simulink model "inertia_sensor"  (R2024b)
settings: Solver=VariableStepAuto  StartTime=0.0  StopTime=10.0  RelTol=1e-3
libraries: nesl_utility x7, sm_lib x6
settings Model: Creator=tarak  LastModifiedBy=tarak

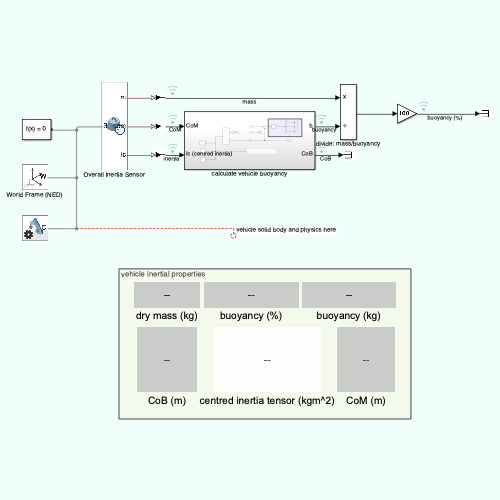
[thumbnail: Simulink's stored preview of the top-level diagram]
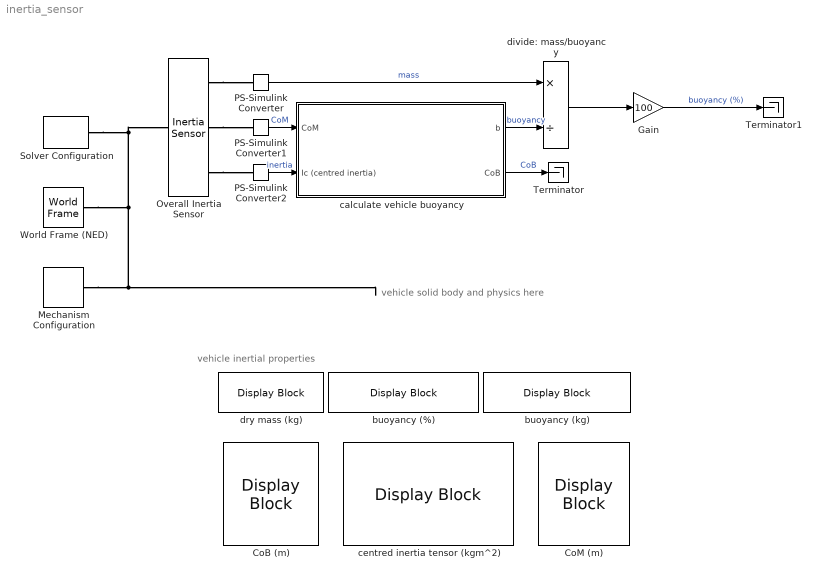
== system inertia_sensor ==
  note: vehicle inertial properties
  note: vehicle solid body and physics here
  CoB (m) : DisplayBlock  LabelPosition=Hide  Transparency=1
  CoM (m) : DisplayBlock  LabelPosition=Hide  Transparency=1
  Gain : Gain  Gain=100
  Mechanism Configuration : sm_lib/Utilities/Mechanism Configuration  UniformGravity=Constant  GravityVector=[0 0 -9.80665]  GravityVectorUnits=m/s^2  LinearizationDelta=0.001  JointModeTransitionNonlinearIterations=2
  Overall Inertia Sensor : sm_lib/Body Elements/Inertia Sensor  SensorExtent=Mechanism  SpanWeldJoints=off  ExcludeGroundedBodies=off  MeasurementFrame=World  SenseMass=on  SenseCenterOfMass=on  SenseInertiaMatrix=off  SenseCenteredInertiaMatrix=on  SensePrincipalInertiaMatrix=off  SenseRotationMatrix=off  GraphicType=PrincipalInertiaFrame  PrincipalInertiaFrameSize=20  GraphicVisPropType=SimpleVisualProperties  GraphicDiffuseColor=[0.5 0.5 0.5]  GraphicOpacity=1  GraphicSpecularColor=[0.5 0.5 0.5 1.0]  GraphicAmbientColor=[0.15 0.15 0.15 1.0]  GraphicEmissiveColor=[0.0 0.0 0.0 1.0]  GraphicShininess=75
  PS-Simulink Converter : nesl_utility/PS-Simulink Converter  PhysicalDomain=network_engine_domain  SubClassName=ps_output  LeftPortType=input  RightPortType=output  PseudoPeriodic=off  Frequencies=[]  VectorFormat=inherit  Unit=inherit  AffineConversion=off
  PS-Simulink Converter1 : nesl_utility/PS-Simulink Converter  PhysicalDomain=network_engine_domain  SubClassName=ps_output  LeftPortType=input  RightPortType=output  PseudoPeriodic=off  Frequencies=[]  VectorFormat=inherit  Unit=inherit  AffineConversion=off
  PS-Simulink Converter2 : nesl_utility/PS-Simulink Converter  PhysicalDomain=network_engine_domain  SubClassName=ps_output  LeftPortType=input  RightPortType=output  PseudoPeriodic=off  Frequencies=[]  VectorFormat=inherit  Unit=inherit  AffineConversion=off
  Solver Configuration : nesl_utility/Solver Configuration  PhysicalDomain=network_engine_domain  SubClassName=solver  LeftPortType=input  RightPortType=generic  Tones=[]  Harmonics=[]  SimulateNoise=off  Profile=off  UseLocalSampling=off  EnableSwitchedLinearOptims=on  FrequencyDomain=off  UseCCode=off  RelTol=0.001  AbsTol=0.001  MinStep=1e-09  ToWorkspace=off  RevertToSquareIcSolve=off  NumHomotopyIterations=100  PhasorMode=off  PhasorModeNumHarmonics=1  ConsistencySolver=NEWTON_XTOL_AFTER_FTOL  IndexReductionMethod=DerivativeReplacement  DoDC=off  ResidualTolerance=1e-09  ConsistencyTolSource=GLOBAL  ConsistencyAbsTol=0.001  ConsistencyRelTol=0.001  ConsistencyTolFactor=0.001  UseLocalSolver=off  LocalSolverChoice=NE_BACKWARD_EULER_ADVANCER  ResolveIndetEquations=on  FunctionEvalNumThread=1  LocalSolverSampleTime=0.001  DoFixedCost=off  MaxNonlinIter=3  MaxModeIter=2  ComputeImpulses=off  ImpulseIterations=2  LinearAlgebra=auto  LinearAlgebraNumThread=0  EquationFormulation=NE_TIME_EF  DelaysMemoryBudget=1024  AutomaticFiltering=on  FilteringTimeConstant=0.001  PartitionStorageMethod=AS_NEEDED  PartitionMemoryBudget=1024  PartitionMethod=ROBUST  MultibodyUseLocalSolver=off  MultibodyLocalSolverChoice=ODE1  MultibodyLocalSolverSampleTime=0.001
  Terminator : Terminator
  Terminator1 : Terminator
  World Frame (NED) : sm_lib/Frames and Transforms/World Frame
  buoyancy (%) : DisplayBlock  LabelPosition=Hide  Transparency=1
  buoyancy (kg) : DisplayBlock  LabelPosition=Hide  Transparency=1
  calculate vehicle buoyancy : Subsystem
  centred inertia tensor (kgm^2) : DisplayBlock  LabelPosition=Hide  Transparency=1
  divide: mass/buoyancy : Product  Inputs=*/
  dry mass (kg) : DisplayBlock  LabelPosition=Hide  Transparency=1
  wires:
  PS-Simulink Converter/1 -> divide: mass/buoyancy/1  "mass"
  divide: mass/buoyancy/1 -> Gain/1
  PS-Simulink Converter1/1 -> calculate vehicle buoyancy/1(CoM)  "CoM"
  PS-Simulink Converter2/1 -> calculate vehicle buoyancy/2(Ic (centred inertia))  "inertia"
  calculate vehicle buoyancy/1(b) -> divide: mass/buoyancy/2  "buoyancy"
  calculate vehicle buoyancy/2(CoB) -> Terminator/1  "CoB"
  Gain/1 -> Terminator1/1  "buoyancy (%)"
  connections:
  Overall Inertia Sensor/RConn3 -- PS-Simulink Converter2/LConn1
  Overall Inertia Sensor/RConn2 -- PS-Simulink Converter1/LConn1
  Overall Inertia Sensor/RConn1 -- PS-Simulink Converter/LConn1
  Solver Configuration/RConn1 -- Mechanism Configuration/RConn1 -- World Frame (NED)/RConn1 -- Overall Inertia Sensor/LConn1

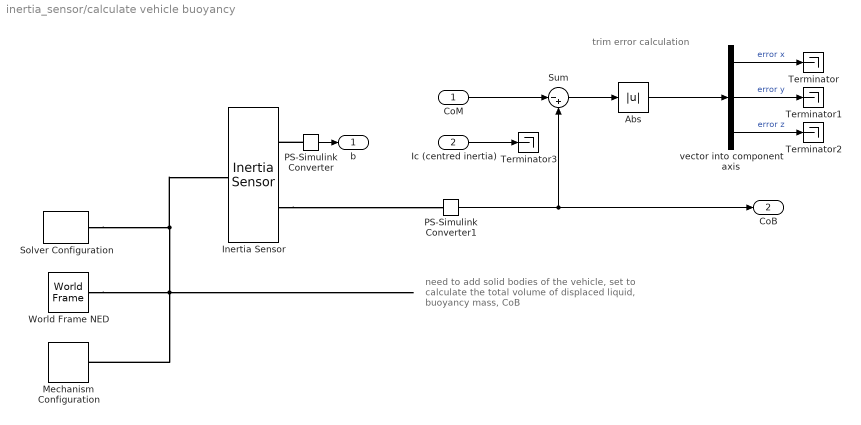
== system inertia_sensor/calculate vehicle buoyancy ==
  note: need to add solid bodies of the vehicle, set to calculate the total volume of displaced liquid, buoyancy mass, CoB
  note: trim error calculation
  CoM : Inport
  Ic (centred inertia) : Inport  Port=2
  Abs : Abs  SaturateOnIntegerOverflow=off
  Inertia Sensor : sm_lib/Body Elements/Inertia Sensor  SensorExtent=Mechanism  SpanWeldJoints=off  ExcludeGroundedBodies=off  MeasurementFrame=World  SenseMass=on  SenseCenterOfMass=on  SenseInertiaMatrix=off  SenseCenteredInertiaMatrix=off  SensePrincipalInertiaMatrix=off  SenseRotationMatrix=off  GraphicType=PrincipalInertiaFrame  PrincipalInertiaFrameSize=20  GraphicVisPropType=SimpleVisualProperties  GraphicDiffuseColor=[0.5 0.5 0.5]  GraphicOpacity=1  GraphicSpecularColor=[0.5 0.5 0.5 1.0]  GraphicAmbientColor=[0.15 0.15 0.15 1.0]  GraphicEmissiveColor=[0.0 0.0 0.0 1.0]  GraphicShininess=75
  Mechanism Configuration : sm_lib/Utilities/Mechanism Configuration  UniformGravity=Constant  GravityVector=[0 0 -9.80665]  GravityVectorUnits=m/s^2  LinearizationDelta=0.001  JointModeTransitionNonlinearIterations=2
  PS-Simulink Converter : nesl_utility/PS-Simulink Converter  PhysicalDomain=network_engine_domain  SubClassName=ps_output  LeftPortType=input  RightPortType=output  PseudoPeriodic=off  Frequencies=[]  VectorFormat=inherit  Unit=inherit  AffineConversion=off
  PS-Simulink Converter1 : nesl_utility/PS-Simulink Converter  PhysicalDomain=network_engine_domain  SubClassName=ps_output  LeftPortType=input  RightPortType=output  PseudoPeriodic=off  Frequencies=[]  VectorFormat=inherit  Unit=inherit  AffineConversion=off
  Solver Configuration : nesl_utility/Solver Configuration  PhysicalDomain=network_engine_domain  SubClassName=solver  LeftPortType=input  RightPortType=generic  Tones=[]  Harmonics=[]  SimulateNoise=off  Profile=off  UseLocalSampling=off  EnableSwitchedLinearOptims=on  FrequencyDomain=off  UseCCode=off  RelTol=0.001  AbsTol=0.001  MinStep=1e-09  ToWorkspace=off  RevertToSquareIcSolve=off  NumHomotopyIterations=100  PhasorMode=off  PhasorModeNumHarmonics=1  ConsistencySolver=NEWTON_XTOL_AFTER_FTOL  IndexReductionMethod=DerivativeReplacement  DoDC=off  ResidualTolerance=1e-09  ConsistencyTolSource=GLOBAL  ConsistencyAbsTol=0.001  ConsistencyRelTol=0.001  ConsistencyTolFactor=0.001  UseLocalSolver=off  LocalSolverChoice=NE_BACKWARD_EULER_ADVANCER  ResolveIndetEquations=on  FunctionEvalNumThread=1  LocalSolverSampleTime=0.001  DoFixedCost=off  MaxNonlinIter=3  MaxModeIter=2  ComputeImpulses=off  ImpulseIterations=2  LinearAlgebra=auto  LinearAlgebraNumThread=0  EquationFormulation=NE_TIME_EF  DelaysMemoryBudget=1024  AutomaticFiltering=on  FilteringTimeConstant=0.001  PartitionStorageMethod=AS_NEEDED  PartitionMemoryBudget=1024  PartitionMethod=ROBUST  MultibodyUseLocalSolver=off  MultibodyLocalSolverChoice=ODE1  MultibodyLocalSolverSampleTime=0.001
  Sum : Sum  Inputs=|-+
  Terminator{,1..3} (4 alike) : Terminator
  World Frame NED : sm_lib/Frames and Transforms/World Frame
  vector into component axis : Demux  Outputs=3
  b : Outport
  CoB : Outport  Port=2
  wires:
  CoM/1 -> Sum/1
  Sum/1 -> Abs/1
  Abs/1 -> vector into component axis/1
  vector into component axis/1 -> Terminator/1  "error x"
  vector into component axis/2 -> Terminator1/1  "error y"
  vector into component axis/3 -> Terminator2/1  "error z"
  Ic (centred inertia)/1 -> Terminator3/1
  PS-Simulink Converter/1 -> b/1
  PS-Simulink Converter1/1 -> Sum/2, CoB/1
  connections:
  PS-Simulink Converter/LConn1 -- Inertia Sensor/RConn1
  Inertia Sensor/RConn2 -- PS-Simulink Converter1/LConn1
  World Frame NED/RConn1 -- Solver Configuration/RConn1 -- Inertia Sensor/LConn1 -- Mechanism Configuration/RConn1
